simulink model "System_with_motor_tf"  (R2018a)
settings: Solver=VariableStepAuto  StartTime=0.0  StopTime=180  RelTol=1e-3
settings Model: Creator=Zeljko  LastModifiedBy=Zeljko

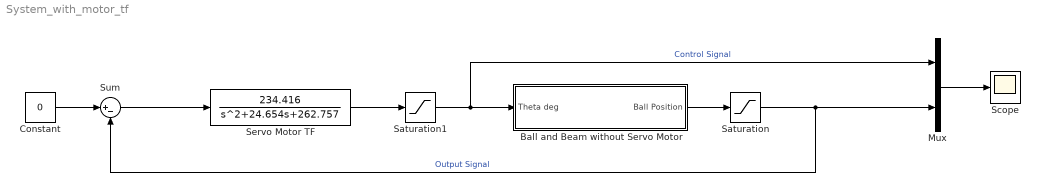
== system System_with_motor_tf ==
  Ball and Beam without Servo Motor : Subsystem
  Constant : Constant  Value=0
  Mux : Mux  Inputs=2
  Saturation : Saturate  UpperLimit=225  LowerLimit=-225
  Saturation1 : Saturate  UpperLimit=30  LowerLimit=-30
  Scope : Scope
  Servo Motor TF : TransferFcn  Numerator=234.416  Denominator=[1 24.654 262.757]
  Sum : Sum  Inputs=|+-
  wires:
  Servo Motor TF/1 -> Saturation1/1
  Constant/1 -> Sum/1
  Ball and Beam without Servo Motor/1(Ball Position) -> Saturation/1
  Saturation/1 -> Mux/2, Sum/2  "Output Signal"
  Sum/1 -> Servo Motor TF/1
  Saturation1/1 -> Mux/1, Ball and Beam without Servo Motor/1(Theta deg)  "Control Signal"
  Mux/1 -> Scope/1

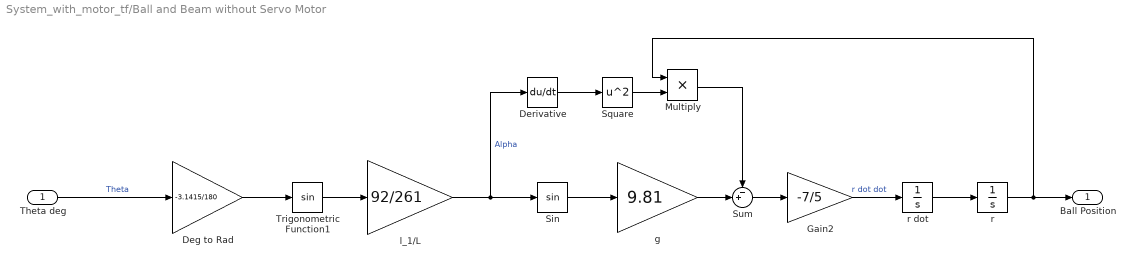
== system System_with_motor_tf/Ball and Beam without Servo Motor ==
  Theta deg : Inport
  Deg to Rad : Gain  Gain=-3.1415/180
  Derivative : Derivative
  Gain2 : Gain  Gain=-7/5
  Multiply : Product
  Sin : Trigonometry
  Square : Math  Operator=square  SaturateOnIntegerOverflow=on
  Sum : Sum  Inputs=-+|
  Trigonometric Function1 : Trigonometry
  g : Gain  Gain=9.81
  l_1/L : Gain  Gain=92/261
  r : Integrator  InitialCondition=100
  r dot : Integrator
  Ball Position : Outport
  wires:
  Theta deg/1 -> Deg to Rad/1  "Theta"
  Deg to Rad/1 -> Trigonometric Function1/1
  r/1 -> Ball Position/1, Multiply/1
  Trigonometric Function1/1 -> l_1/L/1
  l_1/L/1 -> Derivative/1, Sin/1  "Alpha"
  Square/1 -> Multiply/2
  Gain2/1 -> r dot/1  "r dot dot"
  r dot/1 -> r/1
  Derivative/1 -> Square/1
  Multiply/1 -> Sum/1
  g/1 -> Sum/2
  Sum/1 -> Gain2/1
  Sin/1 -> g/1
